simulink library "robot2"
libraries: AtomicLibrary x3, BusImpl x1

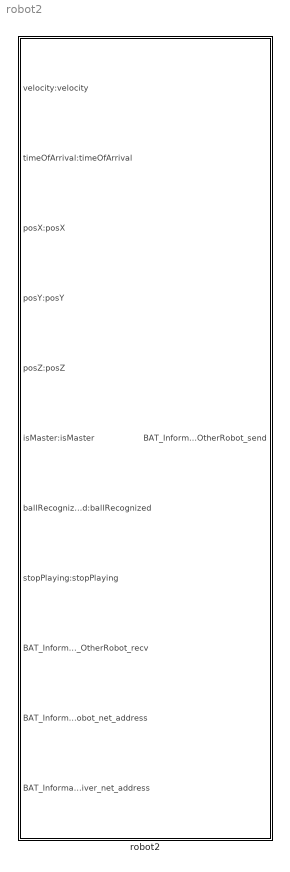
== system robot2 ==
  robot2 : Subsystem  Tag=id=_2Ch5EKbHEeKVjd_905naCg

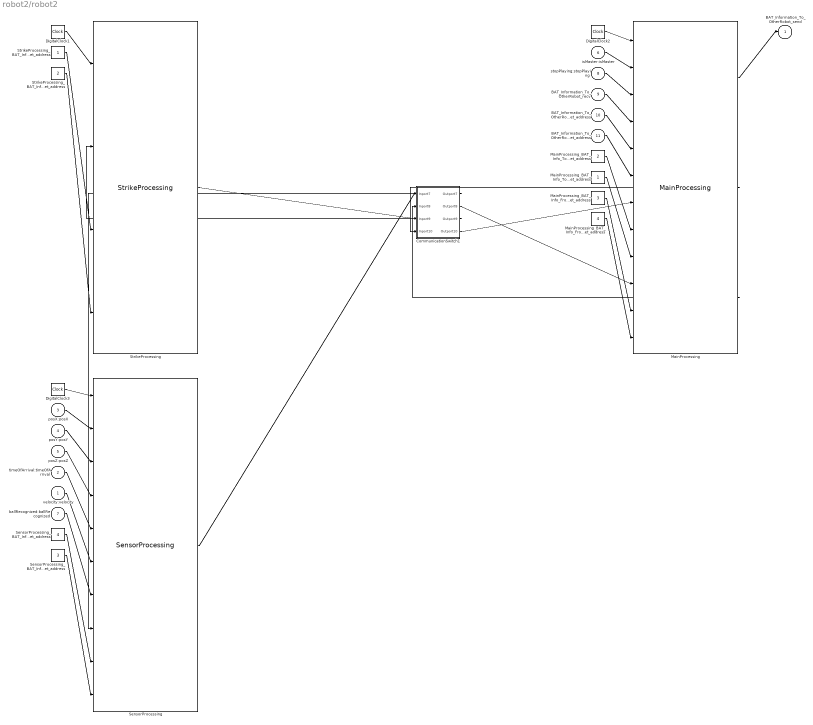
== system robot2/robot2 ==
  velocity:velocity : Inport  Tag=id=_3IbxMKbHEeKVjd_905naCg  Port=1  DataType=double  OutDataType=fixdt(1, 16)  OutScaling=2^0  OutDataTypeStr=double
  timeOfArrival:timeOfArrival : Inport  Tag=id=_3IusIKbHEeKVjd_905naCg  Port=2  DataType=double  OutDataType=fixdt(1, 16)  OutScaling=2^0  OutDataTypeStr=double
  posX:posX : Inport  Tag=id=_3JQQkKbHEeKVjd_905naCg  Port=3  DataType=double  OutDataType=fixdt(1, 16)  OutScaling=2^0  OutDataTypeStr=double
  posY:posY : Inport  Tag=id=_3J3UkKbHEeKVjd_905naCg  Port=4  DataType=double  OutDataType=fixdt(1, 16)  OutScaling=2^0  OutDataTypeStr=double
  posZ:posZ : Inport  Tag=id=_3KbVQKbHEeKVjd_905naCg  Port=5  DataType=double  OutDataType=fixdt(1, 16)  OutScaling=2^0  OutDataTypeStr=double
  isMaster:isMaster : Inport  Tag=id=_3K2zEKbHEeKVjd_905naCg  Port=6  DataType=boolean  OutDataType=fixdt(1, 16)  OutScaling=2^0  OutDataTypeStr=boolean
  ballRecognized:ballRecognized : Inport  Tag=id=_3LazwKbHEeKVjd_905naCg  Port=7  DataType=boolean  OutDataType=fixdt(1, 16)  OutScaling=2^0  OutDataTypeStr=boolean
  stopPlaying:stopPlaying : Inport  Tag=id=_3L1DcKbHEeKVjd_905naCg  Port=8  DataType=boolean  OutDataType=fixdt(1, 16)  OutScaling=2^0  OutDataTypeStr=boolean
  BAT_Information_To_OtherRobot_recv : Inport  Tag=id=_3M1wEKbHEeKVjd_905naCg  Port=9  DataType=auto  OutDataType=fixdt(1, 16)  OutScaling=2^0  UseBusObject=on  OutDataTypeStr=Inherit: auto
      settings: BusObject=PacketBus
  BAT_Information_To_OtherRobot_net_address : Inport  Tag=id=_3M2XIKbHEeKVjd_905naCg  Port=10  DataType=uint8  OutDataType=fixdt(1, 16)  OutScaling=2^0  OutDataTypeStr=uint8
  BAT_Information_To_OtherRobot_receiver_net_address : Inport  Tag=id=_3M2-MKbHEeKVjd_905naCg  Port=11  DataType=uint8  OutDataType=fixdt(1, 16)  OutScaling=2^0  OutDataTypeStr=uint8
  BAT_Information_To_OtherRobot_send : Outport  Tag=id=_3M1wEabHEeKVjd_905naCg  Port=1  DataType=auto  OutDataType=fixdt(1, 16)  OutScaling=2^0  UseBusObject=on  OutDataTypeStr=Inherit: auto
      settings: BusObject=PacketBus
  CommunicationSwitch1 : Subsystem  Tag=id=_2CigIKbHEeKVjd_905naCg  LoadFcn=MainBusGenerator
  StrikeProcessing : AtomicLibrary/StrikeProcessing  Tag=id=_2E6esKbHEeKVjd_905naCg
  DigitalClock1 : DigitalClock  Tag=id=_2E7FwKbHEeKVjd_905naCg  SampleTime=0.0010
  MainProcessing : AtomicLibrary/MainProcessing  Tag=id=_2E_XMKbHEeKVjd_905naCg
  DigitalClock2 : DigitalClock  Tag=id=_2E_-QKbHEeKVjd_905naCg  SampleTime=0.0010
  SensorProcessing : AtomicLibrary/SensorProcessing  Tag=id=_2FGE4KbHEeKVjd_905naCg
  DigitalClock3 : DigitalClock  Tag=id=_2FHTAKbHEeKVjd_905naCg  SampleTime=0.0010
  StrikeProcessing_BAT_Info1_net_address : Constant  Tag=id=_3DME0KbHEeKVjd_905naCg  Value=1  OutDataTypeMode=uint8  OutDataTypeStr=uint8
  MainProcessing_BAT_Info_ToStrikeProcessing1_net_address : Constant  Tag=id=_3DdxoKbHEeKVjd_905naCg  Value=2  OutDataTypeMode=uint8  OutDataTypeStr=uint8
  MainProcessing_BAT_Info_From_SensorProcessing1_net_address : Constant  Tag=id=_3DvecKbHEeKVjd_905naCg  Value=3  OutDataTypeMode=uint8  OutDataTypeStr=uint8
  SensorProcessing_BAT_Info1_net_address : Constant  Tag=id=_3EKVMKbHEeKVjd_905naCg  Value=4  OutDataTypeMode=uint8  OutDataTypeStr=uint8
  SensorProcessing_BAT_Info1_receiver_net_address : Constant  Tag=id=_4y2EkqbHEeKVjd_905naCg  Value=3  OutDataTypeMode=uint8  OutDataTypeStr=uint8
  MainProcessing_BAT_Info_From_SensorProcessing1_receiver_net_address : Constant  Tag=id=_4y3SsKbHEeKVjd_905naCg  Value=4  OutDataTypeMode=uint8  OutDataTypeStr=uint8
  StrikeProcessing_BAT_Info1_receiver_net_address : Constant  Tag=id=_4y_1labHEeKVjd_905naCg  Value=2  OutDataTypeMode=uint8  OutDataTypeStr=uint8
  MainProcessing_BAT_Info_ToStrikeProcessing1_receiver_net_address : Constant  Tag=id=_4zBDsabHEeKVjd_905naCg  Value=1  OutDataTypeMode=uint8  OutDataTypeStr=uint8
  wires:
  DigitalClock1/1 -> StrikeProcessing/1
  DigitalClock2/1 -> MainProcessing/1
  DigitalClock3/1 -> SensorProcessing/1
  StrikeProcessing_BAT_Info1_net_address/1 -> StrikeProcessing/3
  MainProcessing_BAT_Info_ToStrikeProcessing1_net_address/1 -> MainProcessing/8
  MainProcessing_BAT_Info_From_SensorProcessing1_net_address/1 -> MainProcessing/11
  SensorProcessing_BAT_Info1_net_address/1 -> SensorProcessing/9
  SensorProcessing/1 -> CommunicationSwitch1/1(Inport7)
  MainProcessing/3 -> CommunicationSwitch1/2(Inport8)
  CommunicationSwitch1/2(Outport8) -> MainProcessing/10
  CommunicationSwitch1/1(Outport7) -> SensorProcessing/8
  SensorProcessing_BAT_Info1_receiver_net_address/1 -> SensorProcessing/10
  MainProcessing_BAT_Info_From_SensorProcessing1_receiver_net_address/1 -> MainProcessing/12
  StrikeProcessing/1 -> CommunicationSwitch1/3(Inport9)
  MainProcessing/2 -> CommunicationSwitch1/4(Inport10)
  CommunicationSwitch1/4(Outport10) -> MainProcessing/7
  CommunicationSwitch1/3(Outport9) -> StrikeProcessing/2
  StrikeProcessing_BAT_Info1_receiver_net_address/1 -> StrikeProcessing/4
  MainProcessing_BAT_Info_ToStrikeProcessing1_receiver_net_address/1 -> MainProcessing/9
  isMaster:isMaster/1 -> MainProcessing/2
  stopPlaying:stopPlaying/1 -> MainProcessing/3
  ballRecognized:ballRecognized/1 -> SensorProcessing/7
  velocity:velocity/1 -> SensorProcessing/6
  posY:posY/1 -> SensorProcessing/3
  timeOfArrival:timeOfArrival/1 -> SensorProcessing/5
  posX:posX/1 -> SensorProcessing/2
  posZ:posZ/1 -> SensorProcessing/4
  BAT_Information_To_OtherRobot_recv/1 -> MainProcessing/4
  MainProcessing/1 -> BAT_Information_To_OtherRobot_send/1
  BAT_Information_To_OtherRobot_receiver_net_address/1 -> MainProcessing/6
  BAT_Information_To_OtherRobot_net_address/1 -> MainProcessing/5

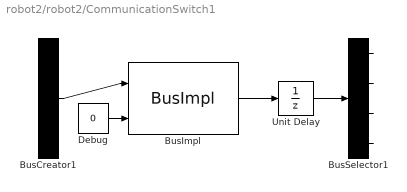
== system robot2/robot2/CommunicationSwitch1 ==
  Inport7 : Inport  Tag=id=_4y35wKbHEeKVjd_905naCg  Port=1  DataType=auto  OutDataType=fixdt(1, 16)  OutScaling=2^0  UseBusObject=on  OutDataTypeStr=Inherit: auto
      settings: BusObject=PacketBus
  Inport8 : Inport  Tag=id=_4y35wqbHEeKVjd_905naCg  Port=2  DataType=auto  OutDataType=fixdt(1, 16)  OutScaling=2^0  UseBusObject=on  OutDataTypeStr=Inherit: auto
      settings: BusObject=PacketBus
  Inport9 : Inport  Tag=id=_4zBqwKbHEeKVjd_905naCg  Port=3  DataType=auto  OutDataType=fixdt(1, 16)  OutScaling=2^0  UseBusObject=on  OutDataTypeStr=Inherit: auto
      settings: BusObject=PacketBus
  Inport10 : Inport  Tag=id=_4zCR0abHEeKVjd_905naCg  Port=4  DataType=auto  OutDataType=fixdt(1, 16)  OutScaling=2^0  UseBusObject=on  OutDataTypeStr=Inherit: auto
      settings: BusObject=PacketBus
  Outport7 : Outport  Tag=id=_4y35wabHEeKVjd_905naCg  Port=1  DataType=auto  OutDataType=fixdt(1, 16)  OutScaling=2^0  UseBusObject=on  OutDataTypeStr=Inherit: auto
      settings: BusObject=PacketBus
  Outport8 : Outport  Tag=id=_4y4g0KbHEeKVjd_905naCg  Port=2  DataType=auto  OutDataType=fixdt(1, 16)  OutScaling=2^0  UseBusObject=on  OutDataTypeStr=Inherit: auto
      settings: BusObject=PacketBus
  Outport9 : Outport  Tag=id=_4zCR0KbHEeKVjd_905naCg  Port=3  DataType=auto  OutDataType=fixdt(1, 16)  OutScaling=2^0  UseBusObject=on  OutDataTypeStr=Inherit: auto
      settings: BusObject=PacketBus
  Outport10 : Outport  Tag=id=_4zCR0qbHEeKVjd_905naCg  Port=4  DataType=auto  OutDataType=fixdt(1, 16)  OutScaling=2^0  UseBusObject=on  OutDataTypeStr=Inherit: auto
      settings: BusObject=PacketBus
  BusCreator1 : BusCreator  Inputs=4  UseBusObject=on
      settings: BusObject=MainBus
  BusSelector1 : BusSelector  OutputSignals=rc1,rc2,rc3,rc4
  Unit Delay : UnitDelay  SampleTime=-1
  BusImpl : BusImpl/BusImpl
  Debug : Constant  Value=0  OutDataType=fixdt(1, 16)  OutScaling=2^0
  wires:
  BusImpl/1 -> Unit Delay/1
  BusCreator1/1 -> BusImpl/1
  Unit Delay/1 -> BusSelector1/1
  Inport7/1 -> BusCreator1/1  "rc1"
  Inport8/1 -> BusCreator1/2  "rc2"
  Inport9/1 -> BusCreator1/3  "rc3"
  Inport10/1 -> BusCreator1/4  "rc4"
  BusSelector1/1 -> Outport7/1
  BusSelector1/2 -> Outport8/1
  BusSelector1/3 -> Outport9/1
  BusSelector1/4 -> Outport10/1
  Debug/1 -> BusImpl/2
